simulink model "Simulink"  (R2020b)
settings: Solver=VariableStepAuto  StartTime=0.0  StopTime=11.2395  RelTol=1e-3
values from neighbouring files (symbols this model uses):
  alpha_0 = 1    [Main.m]
  b = 10    [Main.m]
  beta = 3    [Main.m]
  beta_0 = 1    [Main.m]
  c1 = rand(8,8)-0.5    [Main.m]
  c2 = rand(8,8)-0.5    [Main.m]
  c3 = rand(8,8)-0.5    [Main.m]
  c4 = rand(8,8)-0.5    [Main.m]
  delta_0 = 1    [Main.m]
  Gamma = 3    [Main.m]
  gamma = 0.1    [Main.m]
  h1_x = 5    [Main.m]
  h1_y = 5    [Main.m]
  h2_x = -5    [Main.m]
  h2_y = 5    [Main.m]
  h3_x = -5    [Main.m]
  h3_y = -5    [Main.m]
  h4_x = 5    [Main.m]
  h4_y = -5    [Main.m]
  kapa = 3    [Main.m]
  ki = diag([150,150])    [Main.m]
  kp = 20    [Main.m]
  L = full(laplacian(G))    [Main.m]
  m = 3    [Main.m]
  obs_x = 40    [Main.m]
  obs_y = 0    [Main.m]
  R = 5    [Main.m]
  r = 2    [Main.m]
  R_reg = 15    [Main.m]
  region_x = 80    [Main.m]
  region_y = 0    [Main.m]
  row_0 = 0    [Main.m]
  WL_0 = rand(number_of_neurons,1)*2    [Main.m]
  WR_0 = rand(number_of_neurons,1)*2    [Main.m]
  x1_0 = 1    [Main.m]
  x1_dot_0 = 0    [Main.m]
  x2_0 = 1    [Main.m]
  x2_dot_0 = 0    [Main.m]
  x3_0 = 1    [Main.m]
  x3_dot_0 = 0    [Main.m]
  x4_0 = 1    [Main.m]
  x4_dot_0 = 0    [Main.m]
  y1_0 = 9    [Main.m]
  y1_dot_0 = 0    [Main.m]
  y2_0 = 3    [Main.m]
  y2_dot_0 = 0    [Main.m]
  y3_0 = -3    [Main.m]
  y3_dot_0 = 0    [Main.m]
  y4_0 = -9    [Main.m]
  y4_dot_0 = 0    [Main.m]
(part 1 of 2)
settings Model: Creator=sokra  LastModifiedBy=sokra

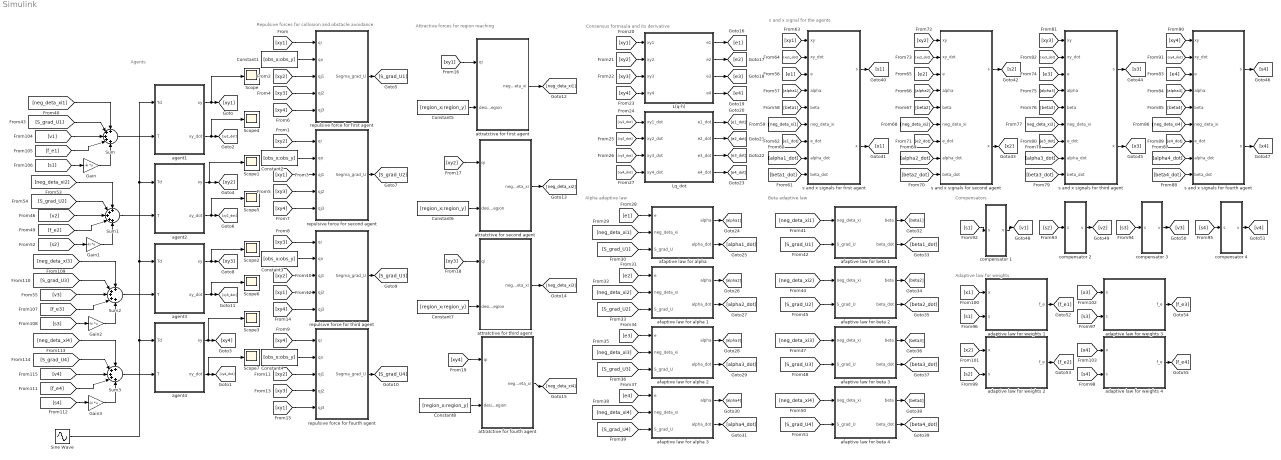
== system Simulink ==
  note: Adaptive law for weights
  note: Compensators
  note: s and x signal for the agents
  note: Alpha adaptive law
  note: Consensus formaula and its derivative
  note: Attractive forces for region reaching
  note: Repulsive forces for collosion and obstacle avoidance
  note: Agents
  note: Beta adaptive law
  Constant{1..4} (4 alike) : Constant  Value=[obs_x;obs_y]
  Constant{5..8} (4 alike) : Constant  Value=[region_x;region_y]
  Gain{,1..3} (4 alike) : Gain  Gain=-ki  Multiplication=Matrix(K*u)
  L(q-h) : Subsystem
  Lq_dot : Subsystem
  Scope{,1..7} (8 alike) : Scope
  Sine Wave : Sin  Amplitude=2  Frequency=[1;2]  Phase=[0;pi/2]  SampleTime=0
  Sum{,1..3} (4 alike) : Sum  Inputs=+++++
  adaptive law for weights 1 : Subsystem  mask{c=c1}
  adaptive law for weights 2 : Subsystem  mask{c=c2}
  adaptive law for weights 3 : Subsystem  mask{c=c3}
  adaptive law for weights 4 : Subsystem  mask{c=c4}
  "afaptive law for alpha " : Subsystem
  afaptive law for alpha 1 : Subsystem
  afaptive law for alpha 2 : Subsystem
  afaptive law for alpha 3 : Subsystem
  afaptive law for beta 1 : Subsystem
  afaptive law for beta 2 : Subsystem
  afaptive law for beta 3 : Subsystem
  afaptive law for beta 4 : Subsystem
  agent1 : Subsystem  mask{agent_x_0=x1_0, agent_y_0=y1_0, agent_x_dot_0=x1_dot_0, agent_y_dot_0=y1_dot_0}
  agent2 : Subsystem  mask{agent_x_0=x2_0, agent_y_0=y2_0, agent_x_dot_0=x2_dot_0, agent_y_dot_0=y2_dot_0}
  agent3 : Subsystem  mask{agent_x_0=x3_0, agent_y_0=y3_0, agent_x_dot_0=x3_dot_0, agent_y_dot_0=y3_dot_0}
  agent4 : Subsystem  mask{agent_x_0=x4_0, agent_y_0=y4_0, agent_x_dot_0=x4_dot_0, agent_y_dot_0=y4_dot_0}
  attratctive for first agent : Subsystem
  attratctive for fourth agent : Subsystem
  attratctive for second agent : Subsystem
  attratctive for third agent : Subsystem
  compensator 1 : Subsystem
  compensator 2 : Subsystem
  compensator 3 : Subsystem
  compensator 4 : Subsystem
  repulsive force for first agent : Subsystem
  repulsive force for fourth agent : Subsystem
  repulsive force for second agent : Subsystem
  repulsive force for third agent : Subsystem
  s and x signals for first agent : Subsystem
  s and x signals for fourth agent : Subsystem
  s and x signals for second agent : Subsystem
  s and x signals for third agent : Subsystem
  wires:
  Sine Wave/1 -> agent3/1(Td), agent2/1(Td), agent1/1(Td), agent4/1(Td)
  agent1/1(xy) -> Scope/1, [xy1]
  agent1/2(xy_dot) -> Scope4/1, [xy1_dot]
  agent2/1(xy) -> Scope1/1, [xy2]
  agent2/2(xy_dot) -> Scope5/1, [xy2_dot]
  agent3/1(xy) -> Scope2/1, [xy3]
  agent3/2(xy_dot) -> Scope6/1, [xy3_dot]
  agent4/1(xy) -> Scope3/1, [xy4]
  agent4/2(xy_dot) -> Scope7/1, [xy4_dot]
  [xy1] -> repulsive force for first agent/1(qi)
  Constant1/1 -> repulsive force for first agent/2(qo)
  [xy2] -> repulsive force for first agent/3(qj1)
  [xy3] -> repulsive force for first agent/4(qj2)
  [xy4] -> repulsive force for first agent/5(qj3)
  [xy4] -> repulsive force for second agent/5(qj3)
  [xy3] -> repulsive force for second agent/4(qj2)
  [xy1] -> repulsive force for second agent/3(qj1)
  Constant2/1 -> repulsive force for second agent/2(qo)
  [xy2] -> repulsive force for second agent/1(qi)
  [xy4] -> repulsive force for fourth agent/1(qi)
  Constant4/1 -> repulsive force for fourth agent/2(qo)
  [xy2] -> repulsive force for fourth agent/3(qj1)
  [xy3] -> repulsive force for fourth agent/4(qj2)
  [xy1] -> repulsive force for fourth agent/5(qj3)
  [xy4] -> repulsive force for third agent/5(qj3)
  [xy1] -> repulsive force for third agent/4(qj2)
  [xy2] -> repulsive force for third agent/3(qj1)
  Constant3/1 -> repulsive force for third agent/2(qo)
  [xy3] -> repulsive force for third agent/1(qi)
  repulsive force for first agent/1(Segma_grad_U) -> [S_grad_U1]
  repulsive force for second agent/1(Segma_grad_U) -> [S_grad_U2]
  repulsive force for fourth agent/1(Segma_grad_U) -> [S_grad_U4]
  repulsive force for third agent/1(Segma_grad_U) -> [S_grad_U3]
  attratctive for first agent/1(neg_deta_xi) -> [neg_deta_xi1]
  [xy1] -> attratctive for first agent/1(qi)
  Constant5/1 -> attratctive for first agent/2(desired_region)
  Constant6/1 -> attratctive for second agent/2(desired_region)
  [xy2] -> attratctive for second agent/1(qi)
  attratctive for second agent/1(neg_deta_xi) -> [neg_deta_xi2]
  attratctive for fourth agent/1(neg_deta_xi) -> [neg_deta_xi4]
  [xy4] -> attratctive for fourth agent/1(qi)
  Constant8/1 -> attratctive for fourth agent/2(desired_region)
  Constant7/1 -> attratctive for third agent/2(desired_region)
  [xy3] -> attratctive for third agent/1(qi)
  attratctive for third agent/1(neg_deta_xi) -> [neg_deta_xi3]
  [xy1] -> L(q-h)/1(xy1)
  [xy2] -> L(q-h)/2(xy2)
  [xy3] -> L(q-h)/3(xy3)
  [xy4] -> L(q-h)/4(xy4)
  L(q-h)/4(e4) -> [e4]
  L(q-h)/3(e3) -> [e3]
  L(q-h)/2(e2) -> [e2]
  L(q-h)/1(e1) -> [e1]
  Lq_dot/1(e1_dot) -> [e1_dot]
  Lq_dot/2(e2_dot) -> [e2_dot]
  Lq_dot/3(e3_dot) -> [e3_dot]
  Lq_dot/4(e4_dot) -> [e4_dot]
  [xy4_dot] -> Lq_dot/4(xy4_dot)
  [xy3_dot] -> Lq_dot/3(xy3_dot)
  [xy2_dot] -> Lq_dot/2(xy2_dot)
  [xy1_dot] -> Lq_dot/1(xy1_dot)
  [e1] -> "afaptive law for alpha "/1(e)
  [neg_deta_xi1] -> "afaptive law for alpha "/2(neg_deta_xi)
  [S_grad_U1] -> "afaptive law for alpha "/3(S_grad_U)
  "afaptive law for alpha "/1(alpha) -> [alpha1]
  "afaptive law for alpha "/2(alpha_dot) -> [alpha1_dot]
  afaptive law for alpha 1/2(alpha_dot) -> [alpha2_dot]
  afaptive law for alpha 1/1(alpha) -> [alpha2]
  [S_grad_U2] -> afaptive law for alpha 1/3(S_grad_U)
  [neg_deta_xi2] -> afaptive law for alpha 1/2(neg_deta_xi)
  [e2] -> afaptive law for alpha 1/1(e)
  [e3] -> afaptive law for alpha 2/1(e)
  [neg_deta_xi3] -> afaptive law for alpha 2/2(neg_deta_xi)
  [S_grad_U3] -> afaptive law for alpha 2/3(S_grad_U)
  afaptive law for alpha 2/1(alpha) -> [alpha3]
  afaptive law for alpha 2/2(alpha_dot) -> [alpha3_dot]
  afaptive law for alpha 3/2(alpha_dot) -> [alpha4_dot]
  afaptive law for alpha 3/1(alpha) -> [alpha4]
  [S_grad_U4] -> afaptive law for alpha 3/3(S_grad_U)
  [neg_deta_xi4] -> afaptive law for alpha 3/2(neg_deta_xi)
  [e4] -> afaptive law for alpha 3/1(e)
  [neg_deta_xi4] -> afaptive law for beta 4/1(neg_deta_xi)
  [S_grad_U4] -> afaptive law for beta 4/2(S_grad_U)
  afaptive law for beta 4/1(beta) -> [beta4]
  afaptive law for beta 4/2(beta_dot) -> [beta4_dot]
  afaptive law for beta 3/2(beta_dot) -> [beta3_dot]
  afaptive law for beta 3/1(beta) -> [beta3]
  [S_grad_U3] -> afaptive law for beta 3/2(S_grad_U)
  [neg_deta_xi3] -> afaptive law for beta 3/1(neg_deta_xi)
  [neg_deta_xi2] -> afaptive law for beta 2/1(neg_deta_xi)
  [S_grad_U2] -> afaptive law for beta 2/2(S_grad_U)
  afaptive law for beta 2/1(beta) -> [beta2]
  afaptive law for beta 2/2(beta_dot) -> [beta2_dot]
  afaptive law for beta 1/2(beta_dot) -> [beta1_dot]
  afaptive law for beta 1/1(beta) -> [beta1]
  [S_grad_U1] -> afaptive law for beta 1/2(S_grad_U)
  [neg_deta_xi1] -> afaptive law for beta 1/1(neg_deta_xi)
  Sum/1 -> agent1/2(T)
  s and x signals for first agent/2(x) -> [x1]
  s and x signals for first agent/1(s) -> [s1]
  [xy1] -> s and x signals for first agent/1(xy)
  [xy1_dot] -> s and x signals for first agent/2(xy_dot)
  [e1] -> s and x signals for first agent/3(e)
  [alpha1] -> s and x signals for first agent/4(alpha)
  [beta1] -> s and x signals for first agent/5(beta)
  [neg_deta_xi1] -> s and x signals for first agent/6(neg_deta_xi)
  [e1_dot] -> s and x signals for first agent/7(e_dot)
  [alpha1_dot] -> s and x signals for first agent/8(alpha_dot)
  [beta1_dot] -> s and x signals for first agent/9(beta_dot)
  [beta2_dot] -> s and x signals for second agent/9(beta_dot)
  [alpha2_dot] -> s and x signals for second agent/8(alpha_dot)
  [e2_dot] -> s and x signals for second agent/7(e_dot)
  [neg_deta_xi2] -> s and x signals for second agent/6(neg_deta_xi)
  [beta2] -> s and x signals for second agent/5(beta)
  [alpha2] -> s and x signals for second agent/4(alpha)
  [e2] -> s and x signals for second agent/3(e)
  [xy2_dot] -> s and x signals for second agent/2(xy_dot)
  [xy2] -> s and x signals for second agent/1(xy)
  s and x signals for second agent/1(s) -> [s2]
  s and x signals for second agent/2(x) -> [x2]
  s and x signals for third agent/2(x) -> [x3]
  s and x signals for third agent/1(s) -> [s3]
  [xy3] -> s and x signals for third agent/1(xy)
  [xy3_dot] -> s and x signals for third agent/2(xy_dot)
  [e3] -> s and x signals for third agent/3(e)
  [alpha3] -> s and x signals for third agent/4(alpha)
  [beta3] -> s and x signals for third agent/5(beta)
  [neg_deta_xi3] -> s and x signals for third agent/6(neg_deta_xi)
  [e3_dot] -> s and x signals for third agent/7(e_dot)
  [alpha3_dot] -> s and x signals for third agent/8(alpha_dot)
  [beta3_dot] -> s and x signals for third agent/9(beta_dot)
  [beta4_dot] -> s and x signals for fourth agent/9(beta_dot)
  [alpha4_dot] -> s and x signals for fourth agent/8(alpha_dot)
  [e4_dot] -> s and x signals for fourth agent/7(e_dot)
  [neg_deta_xi4] -> s and x signals for fourth agent/6(neg_deta_xi)
  [beta4] -> s and x signals for fourth agent/5(beta)
  [alpha4] -> s and x signals for fourth agent/4(alpha)
  [e4] -> s and x signals for fourth agent/3(e)
  [xy4_dot] -> s and x signals for fourth agent/2(xy_dot)
  [xy4] -> s and x signals for fourth agent/1(xy)
  s and x signals for fourth agent/1(s) -> [s4]
  s and x signals for fourth agent/2(x) -> [x4]
  [s1] -> compensator 1/1(s)
  compensator 1/1(v) -> [v1]
  compensator 2/1(v) -> [v2]
  [s2] -> compensator 2/1(s)
  [s3] -> compensator 3/1(s)
  compensator 3/1(v) -> [v3]
  compensator 4/1(v) -> [v4]
  [s4] -> compensator 4/1(s)
  [s4] -> adaptive law for weights 4/2(s)
  [s1] -> adaptive law for weights 1/2(s)
  [s3] -> adaptive law for weights 3/2(s)
  [s2] -> adaptive law for weights 2/2(s)
  [x4] -> adaptive law for weights 4/1(x)
  [x3] -> adaptive law for weights 3/1(x)
  [x2] -> adaptive law for weights 2/1(x)
  [x1] -> adaptive law for weights 1/1(x)
  adaptive law for weights 3/1(f_e) -> [f_e3]
  adaptive law for weights 4/1(f_e) -> [f_e4]
  adaptive law for weights 1/1(f_e) -> [f_e1]
  adaptive law for weights 2/1(f_e) -> [f_e2]
  [s1] -> Gain/1
  [neg_deta_xi1] -> Sum/1
  [S_grad_U1] -> Sum/2
  [v1] -> Sum/3
  [f_e1] -> Sum/4
  Gain/1 -> Sum/5
  Gain1/1 -> Sum1/5
  [f_e2] -> Sum1/4
  [v2] -> Sum1/3
  [S_grad_U2] -> Sum1/2
  [neg_deta_xi2] -> Sum1/1
  [s2] -> Gain1/1
  Sum1/1 -> agent2/2(T)
  Sum2/1 -> agent3/2(T)
  [s3] -> Gain2/1
  [neg_deta_xi3] -> Sum2/1
  [S_grad_U3] -> Sum2/2
  [v3] -> Sum2/3
  [f_e3] -> Sum2/4
  Gain2/1 -> Sum2/5
  Gain3/1 -> Sum3/5
  [f_e4] -> Sum3/4
  [v4] -> Sum3/3
  [S_grad_U4] -> Sum3/2
  [neg_deta_xi4] -> Sum3/1
  [s4] -> Gain3/1
  Sum3/1 -> agent4/2(T)

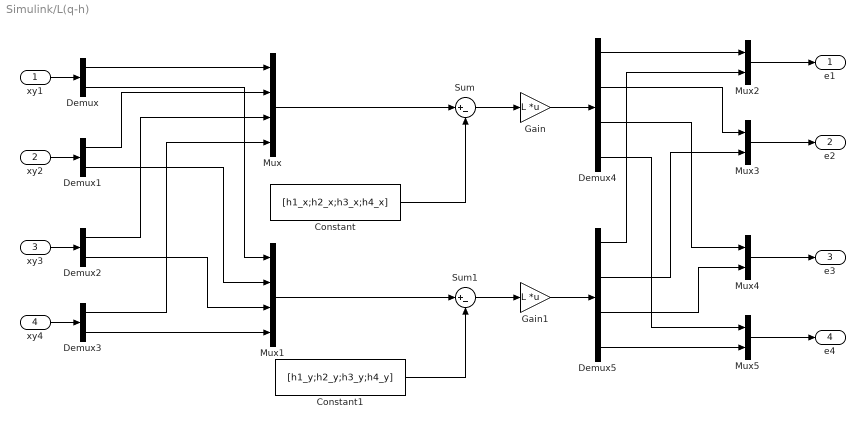
== system Simulink/L(q-h) ==
  xy1 : Inport
  xy2 : Inport  Port=2
  xy3 : Inport  Port=3
  xy4 : Inport  Port=4
  Constant : Constant  Value=[h1_x;h2_x;h3_x;h4_x]
  Constant1 : Constant  Value=[h1_y;h2_y;h3_y;h4_y]
  Demux{,1..3} (4 alike) : Demux  Outputs=2
  Demux4 : Demux
  Demux5 : Demux
  Gain : Gain  Gain=L  Multiplication=Matrix(K*u)
  Gain1 : Gain  Gain=L  Multiplication=Matrix(K*u)
  Mux : Mux
  Mux1 : Mux
  Mux{2..5} (4 alike) : Mux  Inputs=2
  Sum : Sum  Inputs=|+-
  Sum1 : Sum  Inputs=|+-
  e1 : Outport
  e2 : Outport  Port=2
  e3 : Outport  Port=3
  e4 : Outport  Port=4
  wires:
  xy1/1 -> Demux/1
  xy2/1 -> Demux1/1
  xy3/1 -> Demux2/1
  xy4/1 -> Demux3/1
  Demux/1 -> Mux/1
  Demux1/1 -> Mux/2
  Demux2/1 -> Mux/3
  Demux3/1 -> Mux/4
  Demux/2 -> Mux1/1
  Demux1/2 -> Mux1/2
  Demux2/2 -> Mux1/3
  Demux3/2 -> Mux1/4
  Mux/1 -> Sum/1
  Constant/1 -> Sum/2
  Mux1/1 -> Sum1/1
  Constant1/1 -> Sum1/2
  Sum/1 -> Gain/1
  Sum1/1 -> Gain1/1
  Gain/1 -> Demux4/1
  Gain1/1 -> Demux5/1
  Mux5/1 -> e4/1
  Mux4/1 -> e3/1
  Mux3/1 -> e2/1
  Mux2/1 -> e1/1
  Demux4/1 -> Mux2/1
  Demux4/2 -> Mux3/1
  Demux4/3 -> Mux4/1
  Demux4/4 -> Mux5/1
  Demux5/4 -> Mux5/2
  Demux5/3 -> Mux4/2
  Demux5/2 -> Mux3/2
  Demux5/1 -> Mux2/2

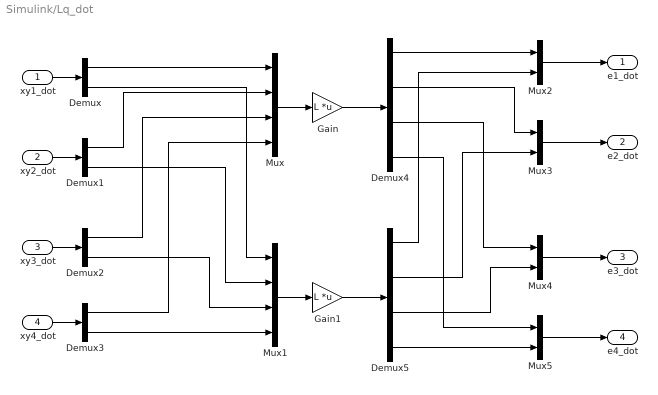
== system Simulink/Lq_dot ==
  xy1_dot : Inport
  xy2_dot : Inport  Port=2
  xy3_dot : Inport  Port=3
  xy4_dot : Inport  Port=4
  Demux{,1..3} (4 alike) : Demux  Outputs=2
  Demux4 : Demux
  Demux5 : Demux
  Gain : Gain  Gain=L  Multiplication=Matrix(K*u)
  Gain1 : Gain  Gain=L  Multiplication=Matrix(K*u)
  Mux : Mux
  Mux1 : Mux
  Mux{2..5} (4 alike) : Mux  Inputs=2
  e1_dot : Outport
  e2_dot : Outport  Port=2
  e3_dot : Outport  Port=3
  e4_dot : Outport  Port=4
  wires:
  Demux5/1 -> Mux2/2
  Demux5/2 -> Mux3/2
  Demux5/3 -> Mux4/2
  Demux5/4 -> Mux5/2
  Demux4/4 -> Mux5/1
  Demux4/3 -> Mux4/1
  Demux4/2 -> Mux3/1
  Demux4/1 -> Mux2/1
  Mux2/1 -> e1_dot/1
  Mux3/1 -> e2_dot/1
  Mux4/1 -> e3_dot/1
  Mux5/1 -> e4_dot/1
  Gain1/1 -> Demux5/1
  Gain/1 -> Demux4/1
  Mux1/1 -> Gain1/1
  Demux3/2 -> Mux1/4
  Demux2/2 -> Mux1/3
  Demux1/2 -> Mux1/2
  Demux/2 -> Mux1/1
  Demux3/1 -> Mux/4
  Demux2/1 -> Mux/3
  Demux1/1 -> Mux/2
  Demux/1 -> Mux/1
  xy4_dot/1 -> Demux3/1
  xy3_dot/1 -> Demux2/1
  xy2_dot/1 -> Demux1/1
  xy1_dot/1 -> Demux/1
  Mux/1 -> Gain/1

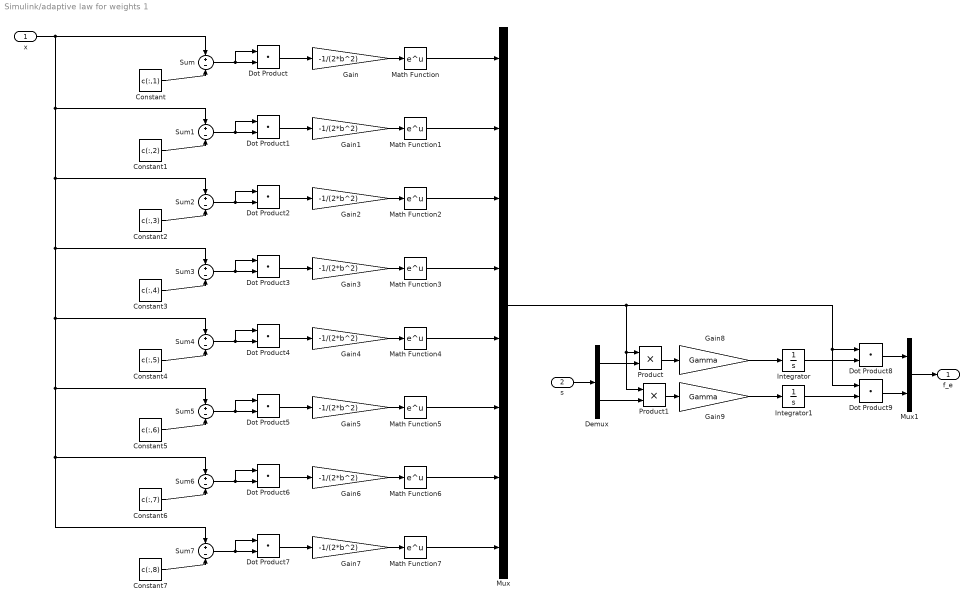
== system Simulink/adaptive law for weights 1 ==
  x : Inport
  s : Inport  Port=2
  Constant : Constant  Value=c(:,1)
  Constant1 : Constant  Value=c(:,2)
  Constant2 : Constant  Value=c(:,3)
  Constant3 : Constant  Value=c(:,4)
  Constant4 : Constant  Value=c(:,5)
  Constant5 : Constant  Value=c(:,6)
  Constant6 : Constant  Value=c(:,7)
  Constant7 : Constant  Value=c(:,8)
  Demux : Demux  Outputs=2
  Dot Product{,1..9} (10 alike) : DotProduct  InputSameDT=on  OutDataTypeStr=Inherit: Inherit via internal rule
  Gain{,1..7} (8 alike) : Gain  Gain=-1/(2*b^2)
  Gain8 : Gain  Gain=Gamma
  Gain9 : Gain  Gain=Gamma
  Integrator : Integrator  InitialCondition=WL_0
  Integrator1 : Integrator  InitialCondition=WR_0
  Math Function{,1..7} (8 alike) : Math  SaturateOnIntegerOverflow=on
  Mux : Mux  Inputs=8
  Mux1 : Mux  Inputs=2
  Product : Product
  Product1 : Product
  Sum{,1..7} (8 alike) : Sum  Inputs=+-
  f_e : Outport
  wires:
  Constant/1 -> Sum/2
  Sum/1 -> Dot Product/2, Dot Product/1
  Dot Product/1 -> Gain/1
  Gain/1 -> Math Function/1
  Math Function/1 -> Mux/1
  Math Function1/1 -> Mux/2
  Gain1/1 -> Math Function1/1
  Dot Product1/1 -> Gain1/1
  Sum1/1 -> Dot Product1/1, Dot Product1/2
  Constant1/1 -> Sum1/2
  Constant2/1 -> Sum2/2
  Sum2/1 -> Dot Product2/2, Dot Product2/1
  Dot Product2/1 -> Gain2/1
  Gain2/1 -> Math Function2/1
  Math Function2/1 -> Mux/3
  Math Function3/1 -> Mux/4
  Gain3/1 -> Math Function3/1
  Dot Product3/1 -> Gain3/1
  Sum3/1 -> Dot Product3/1, Dot Product3/2
  Constant3/1 -> Sum3/2
  Constant4/1 -> Sum4/2
  Sum4/1 -> Dot Product4/2, Dot Product4/1
  Dot Product4/1 -> Gain4/1
  Gain4/1 -> Math Function4/1
  Math Function4/1 -> Mux/5
  Math Function5/1 -> Mux/6
  Gain5/1 -> Math Function5/1
  Dot Product5/1 -> Gain5/1
  Sum5/1 -> Dot Product5/1, Dot Product5/2
  Constant5/1 -> Sum5/2
  Constant6/1 -> Sum6/2
  Sum6/1 -> Dot Product6/2, Dot Product6/1
  Dot Product6/1 -> Gain6/1
  Gain6/1 -> Math Function6/1
  Math Function6/1 -> Mux/7
  Math Function7/1 -> Mux/8
  Gain7/1 -> Math Function7/1
  Dot Product7/1 -> Gain7/1
  Sum7/1 -> Dot Product7/1, Dot Product7/2
  Constant7/1 -> Sum7/2
  x/1 -> Sum7/1, Sum6/1, Sum5/1, Sum4/1, Sum3/1, Sum2/1, Sum1/1, Sum/1
  s/1 -> Demux/1
  Mux/1 -> Dot Product9/1, Dot Product8/1, Product1/1, Product/1
  Demux/1 -> Product/2
  Demux/2 -> Product1/2
  Product/1 -> Gain8/1
  Product1/1 -> Gain9/1
  Gain8/1 -> Integrator/1
  Gain9/1 -> Integrator1/1
  Integrator1/1 -> Dot Product9/2
  Integrator/1 -> Dot Product8/2
  Dot Product8/1 -> Mux1/1
  Dot Product9/1 -> Mux1/2
  Mux1/1 -> f_e/1

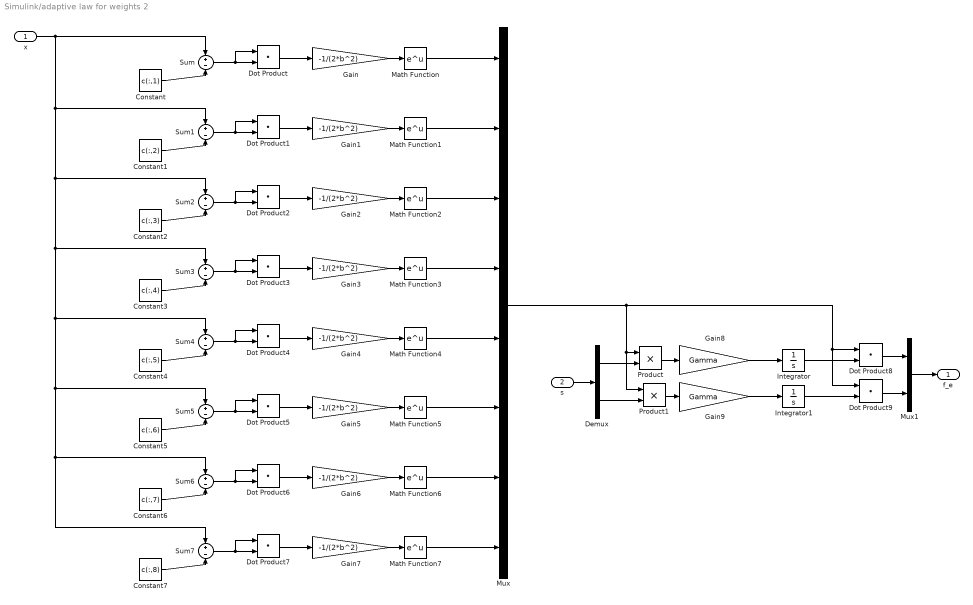
== system Simulink/adaptive law for weights 2 ==
  x : Inport
  s : Inport  Port=2
  Constant : Constant  Value=c(:,1)
  Constant1 : Constant  Value=c(:,2)
  Constant2 : Constant  Value=c(:,3)
  Constant3 : Constant  Value=c(:,4)
  Constant4 : Constant  Value=c(:,5)
  Constant5 : Constant  Value=c(:,6)
  Constant6 : Constant  Value=c(:,7)
  Constant7 : Constant  Value=c(:,8)
  Demux : Demux  Outputs=2
  Dot Product{,1..9} (10 alike) : DotProduct  InputSameDT=on  OutDataTypeStr=Inherit: Inherit via internal rule
  Gain{,1..7} (8 alike) : Gain  Gain=-1/(2*b^2)
  Gain8 : Gain  Gain=Gamma
  Gain9 : Gain  Gain=Gamma
  Integrator : Integrator  InitialCondition=WL_0
  Integrator1 : Integrator  InitialCondition=WR_0
  Math Function{,1..7} (8 alike) : Math  SaturateOnIntegerOverflow=on
  Mux : Mux  Inputs=8
  Mux1 : Mux  Inputs=2
  Product : Product
  Product1 : Product
  Sum{,1..7} (8 alike) : Sum  Inputs=+-
  f_e : Outport
  wires:
  Mux1/1 -> f_e/1
  Gain9/1 -> Integrator1/1
  Dot Product9/1 -> Mux1/2
  Integrator1/1 -> Dot Product9/2
  Math Function3/1 -> Mux/4
  Math Function7/1 -> Mux/8
  Math Function1/1 -> Mux/2
  Math Function5/1 -> Mux/6
  Math Function2/1 -> Mux/3
  Math Function6/1 -> Mux/7
  Constant7/1 -> Sum7/2
  Sum7/1 -> Dot Product7/1, Dot Product7/2
  Dot Product7/1 -> Gain7/1
  Constant3/1 -> Sum3/2
  Sum3/1 -> Dot Product3/1, Dot Product3/2
  Dot Product3/1 -> Gain3/1
  Gain3/1 -> Math Function3/1
  Constant5/1 -> Sum5/2
  Gain5/1 -> Math Function5/1
  Sum1/1 -> Dot Product1/1, Dot Product1/2
  Sum6/1 -> Dot Product6/2, Dot Product6/1
  Dot Product6/1 -> Gain6/1
  Product/1 -> Gain8/1
  Gain/1 -> Math Function/1
  Math Function/1 -> Mux/1
  Constant6/1 -> Sum6/2
  Math Function4/1 -> Mux/5
  Product1/1 -> Gain9/1
  Dot Product4/1 -> Gain4/1
  Sum4/1 -> Dot Product4/2, Dot Product4/1
  Constant4/1 -> Sum4/2
  x/1 -> Sum7/1, Sum6/1, Sum5/1, Sum4/1, Sum3/1, Sum2/1, Sum1/1, Sum/1
  Gain6/1 -> Math Function6/1
  Sum5/1 -> Dot Product5/1, Dot Product5/2
  s/1 -> Demux/1
  Demux/1 -> Product/2
  Mux/1 -> Dot Product9/1, Dot Product8/1, Product1/1, Product/1
  Gain8/1 -> Integrator/1
  Dot Product1/1 -> Gain1/1
  Gain7/1 -> Math Function7/1
  Sum/1 -> Dot Product/2, Dot Product/1
  Dot Product8/1 -> Mux1/1
  Gain1/1 -> Math Function1/1
  Dot Product2/1 -> Gain2/1
  Sum2/1 -> Dot Product2/2, Dot Product2/1
  Gain2/1 -> Math Function2/1
  Demux/2 -> Product1/2
  Constant1/1 -> Sum1/2
  Dot Product/1 -> Gain/1
  Dot Product5/1 -> Gain5/1
  Constant2/1 -> Sum2/2
  Gain4/1 -> Math Function4/1
  Integrator/1 -> Dot Product8/2
  Constant/1 -> Sum/2

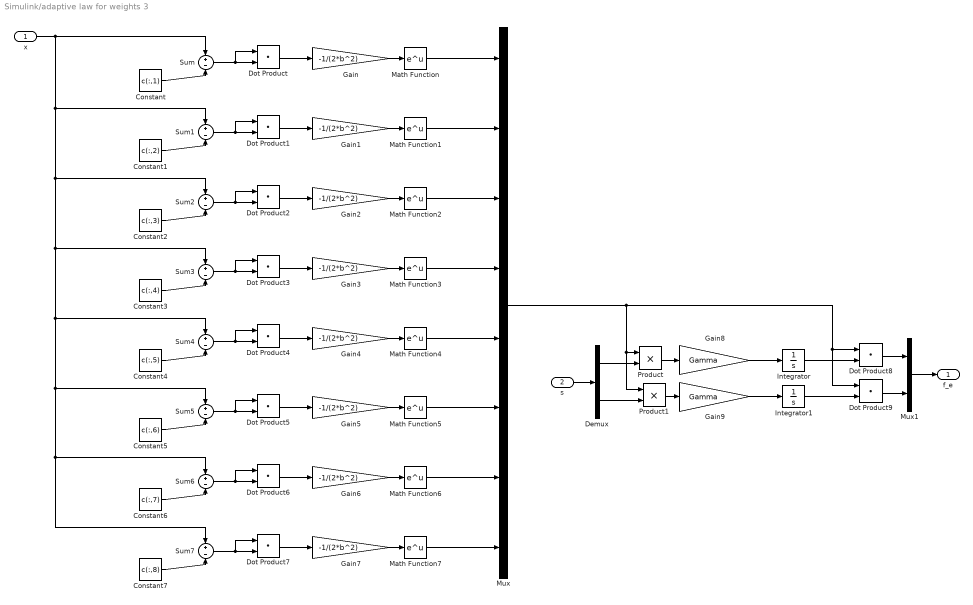
== system Simulink/adaptive law for weights 3 ==
  x : Inport
  s : Inport  Port=2
  Constant : Constant  Value=c(:,1)
  Constant1 : Constant  Value=c(:,2)
  Constant2 : Constant  Value=c(:,3)
  Constant3 : Constant  Value=c(:,4)
  Constant4 : Constant  Value=c(:,5)
  Constant5 : Constant  Value=c(:,6)
  Constant6 : Constant  Value=c(:,7)
  Constant7 : Constant  Value=c(:,8)
  Demux : Demux  Outputs=2
  Dot Product{,1..9} (10 alike) : DotProduct  InputSameDT=on  OutDataTypeStr=Inherit: Inherit via internal rule
  Gain{,1..7} (8 alike) : Gain  Gain=-1/(2*b^2)
  Gain8 : Gain  Gain=Gamma
  Gain9 : Gain  Gain=Gamma
  Integrator : Integrator  InitialCondition=WL_0
  Integrator1 : Integrator  InitialCondition=WR_0
  Math Function{,1..7} (8 alike) : Math  SaturateOnIntegerOverflow=on
  Mux : Mux  Inputs=8
  Mux1 : Mux  Inputs=2
  Product : Product
  Product1 : Product
  Sum{,1..7} (8 alike) : Sum  Inputs=+-
  f_e : Outport
  wires:
  Mux1/1 -> f_e/1
  Gain9/1 -> Integrator1/1
  Dot Product9/1 -> Mux1/2
  Integrator1/1 -> Dot Product9/2
  Math Function3/1 -> Mux/4
  Math Function7/1 -> Mux/8
  Math Function1/1 -> Mux/2
  Math Function5/1 -> Mux/6
  Math Function2/1 -> Mux/3
  Math Function6/1 -> Mux/7
  Constant7/1 -> Sum7/2
  Sum7/1 -> Dot Product7/1, Dot Product7/2
  Dot Product7/1 -> Gain7/1
  Constant3/1 -> Sum3/2
  Sum3/1 -> Dot Product3/1, Dot Product3/2
  Dot Product3/1 -> Gain3/1
  Gain3/1 -> Math Function3/1
  Constant5/1 -> Sum5/2
  Gain5/1 -> Math Function5/1
  Sum1/1 -> Dot Product1/1, Dot Product1/2
  Sum6/1 -> Dot Product6/2, Dot Product6/1
  Dot Product6/1 -> Gain6/1
  Product/1 -> Gain8/1
  Gain/1 -> Math Function/1
  Math Function/1 -> Mux/1
  Constant6/1 -> Sum6/2
  Math Function4/1 -> Mux/5
  Product1/1 -> Gain9/1
  Dot Product4/1 -> Gain4/1
  Sum4/1 -> Dot Product4/2, Dot Product4/1
  Constant4/1 -> Sum4/2
  x/1 -> Sum7/1, Sum6/1, Sum5/1, Sum4/1, Sum3/1, Sum2/1, Sum1/1, Sum/1
  Gain6/1 -> Math Function6/1
  Sum5/1 -> Dot Product5/1, Dot Product5/2
  s/1 -> Demux/1
  Demux/1 -> Product/2
  Mux/1 -> Dot Product9/1, Dot Product8/1, Product1/1, Product/1
  Gain8/1 -> Integrator/1
  Dot Product1/1 -> Gain1/1
  Gain7/1 -> Math Function7/1
  Sum/1 -> Dot Product/2, Dot Product/1
  Dot Product8/1 -> Mux1/1
  Gain1/1 -> Math Function1/1
  Dot Product2/1 -> Gain2/1
  Sum2/1 -> Dot Product2/2, Dot Product2/1
  Gain2/1 -> Math Function2/1
  Demux/2 -> Product1/2
  Constant1/1 -> Sum1/2
  Dot Product/1 -> Gain/1
  Dot Product5/1 -> Gain5/1
  Constant2/1 -> Sum2/2
  Gain4/1 -> Math Function4/1
  Integrator/1 -> Dot Product8/2
  Constant/1 -> Sum/2

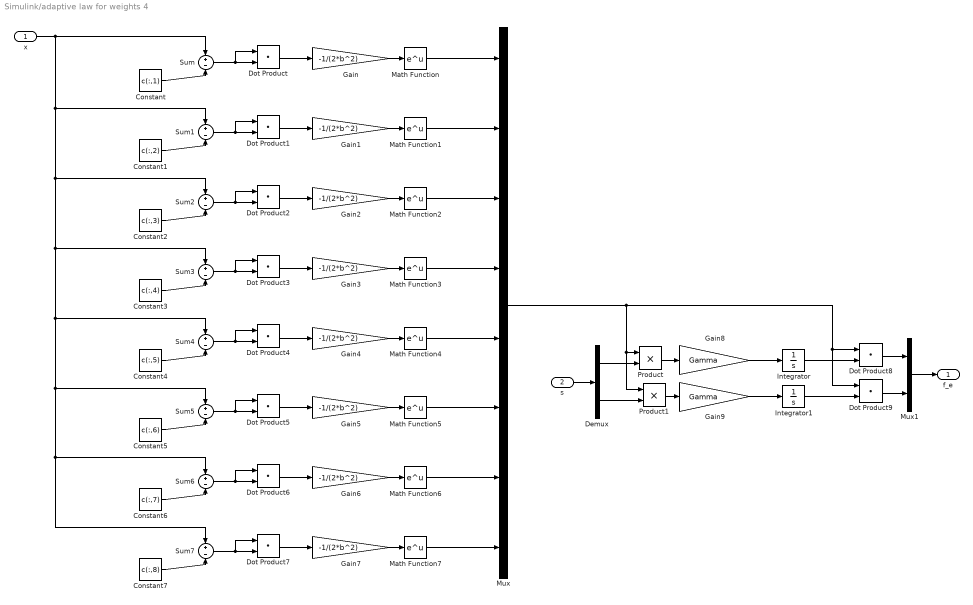
== system Simulink/adaptive law for weights 4 ==
  x : Inport
  s : Inport  Port=2
  Constant : Constant  Value=c(:,1)
  Constant1 : Constant  Value=c(:,2)
  Constant2 : Constant  Value=c(:,3)
  Constant3 : Constant  Value=c(:,4)
  Constant4 : Constant  Value=c(:,5)
  Constant5 : Constant  Value=c(:,6)
  Constant6 : Constant  Value=c(:,7)
  Constant7 : Constant  Value=c(:,8)
  Demux : Demux  Outputs=2
  Dot Product{,1..9} (10 alike) : DotProduct  InputSameDT=on  OutDataTypeStr=Inherit: Inherit via internal rule
  Gain{,1..7} (8 alike) : Gain  Gain=-1/(2*b^2)
  Gain8 : Gain  Gain=Gamma
  Gain9 : Gain  Gain=Gamma
  Integrator : Integrator  InitialCondition=WL_0
  Integrator1 : Integrator  InitialCondition=WR_0
  Math Function{,1..7} (8 alike) : Math  SaturateOnIntegerOverflow=on
  Mux : Mux  Inputs=8
  Mux1 : Mux  Inputs=2
  Product : Product
  Product1 : Product
  Sum{,1..7} (8 alike) : Sum  Inputs=+-
  f_e : Outport
  wires:
  Mux1/1 -> f_e/1
  Gain9/1 -> Integrator1/1
  Dot Product9/1 -> Mux1/2
  Integrator1/1 -> Dot Product9/2
  Math Function3/1 -> Mux/4
  Math Function7/1 -> Mux/8
  Math Function1/1 -> Mux/2
  Math Function5/1 -> Mux/6
  Math Function2/1 -> Mux/3
  Math Function6/1 -> Mux/7
  Constant7/1 -> Sum7/2
  Sum7/1 -> Dot Product7/1, Dot Product7/2
  Dot Product7/1 -> Gain7/1
  Constant3/1 -> Sum3/2
  Sum3/1 -> Dot Product3/1, Dot Product3/2
  Dot Product3/1 -> Gain3/1
  Gain3/1 -> Math Function3/1
  Constant5/1 -> Sum5/2
  Gain5/1 -> Math Function5/1
  Sum1/1 -> Dot Product1/1, Dot Product1/2
  Sum6/1 -> Dot Product6/2, Dot Product6/1
  Dot Product6/1 -> Gain6/1
  Product/1 -> Gain8/1
  Gain/1 -> Math Function/1
  Math Function/1 -> Mux/1
  Constant6/1 -> Sum6/2
  Math Function4/1 -> Mux/5
  Product1/1 -> Gain9/1
  Dot Product4/1 -> Gain4/1
  Sum4/1 -> Dot Product4/2, Dot Product4/1
  Constant4/1 -> Sum4/2
  x/1 -> Sum7/1, Sum6/1, Sum5/1, Sum4/1, Sum3/1, Sum2/1, Sum1/1, Sum/1
  Gain6/1 -> Math Function6/1
  Sum5/1 -> Dot Product5/1, Dot Product5/2
  s/1 -> Demux/1
  Demux/1 -> Product/2
  Mux/1 -> Dot Product9/1, Dot Product8/1, Product1/1, Product/1
  Gain8/1 -> Integrator/1
  Dot Product1/1 -> Gain1/1
  Gain7/1 -> Math Function7/1
  Sum/1 -> Dot Product/2, Dot Product/1
  Dot Product8/1 -> Mux1/1
  Gain1/1 -> Math Function1/1
  Dot Product2/1 -> Gain2/1
  Sum2/1 -> Dot Product2/2, Dot Product2/1
  Gain2/1 -> Math Function2/1
  Demux/2 -> Product1/2
  Constant1/1 -> Sum1/2
  Dot Product/1 -> Gain/1
  Dot Product5/1 -> Gain5/1
  Constant2/1 -> Sum2/2
  Gain4/1 -> Math Function4/1
  Integrator/1 -> Dot Product8/2
  Constant/1 -> Sum/2

== system Simulink/afaptive law for alpha  ==
  e : Inport
  neg_deta_xi : Inport  Port=2
  S_grad_U : Inport  Port=3
  Dot Product : DotProduct  InputSameDT=on  OutDataTypeStr=Inherit: Inherit via internal rule
  Gain : Gain  Gain=-1
  Integrator : Integrator  InitialCondition=alpha_0
  Product : Product
  Sum : Sum
  alpha : Outport
  alpha_dot : Outport  Port=2
  wires:
  Sum/1 -> Dot Product/2
  Product/1 -> Gain/1
  Gain/1 -> alpha_dot/1, Integrator/1
  Dot Product/1 -> Product/1
  S_grad_U/1 -> Sum/2
  e/1 -> Dot Product/1
  neg_deta_xi/1 -> Sum/1
  Integrator/1 -> alpha/1, Product/2

== system Simulink/afaptive law for alpha 1 ==
  e : Inport
  neg_deta_xi : Inport  Port=2
  S_grad_U : Inport  Port=3
  Dot Product : DotProduct  InputSameDT=on  OutDataTypeStr=Inherit: Inherit via internal rule
  Gain : Gain  Gain=-1
  Integrator : Integrator  InitialCondition=alpha_0
  Product : Product
  Sum : Sum
  alpha : Outport
  alpha_dot : Outport  Port=2
  wires:
  Integrator/1 -> Product/2, alpha/1
  neg_deta_xi/1 -> Sum/1
  e/1 -> Dot Product/1
  S_grad_U/1 -> Sum/2
  Dot Product/1 -> Product/1
  Gain/1 -> Integrator/1, alpha_dot/1
  Product/1 -> Gain/1
  Sum/1 -> Dot Product/2

== system Simulink/afaptive law for alpha 2 ==
  e : Inport
  neg_deta_xi : Inport  Port=2
  S_grad_U : Inport  Port=3
  Dot Product : DotProduct  InputSameDT=on  OutDataTypeStr=Inherit: Inherit via internal rule
  Gain : Gain  Gain=-1
  Integrator : Integrator  InitialCondition=alpha_0
  Product : Product
  Sum : Sum
  alpha : Outport
  alpha_dot : Outport  Port=2
  wires:
  Sum/1 -> Dot Product/2
  Product/1 -> Gain/1
  Gain/1 -> alpha_dot/1, Integrator/1
  Dot Product/1 -> Product/1
  S_grad_U/1 -> Sum/2
  e/1 -> Dot Product/1
  neg_deta_xi/1 -> Sum/1
  Integrator/1 -> alpha/1, Product/2

== system Simulink/afaptive law for alpha 3 ==
  e : Inport
  neg_deta_xi : Inport  Port=2
  S_grad_U : Inport  Port=3
  Dot Product : DotProduct  InputSameDT=on  OutDataTypeStr=Inherit: Inherit via internal rule
  Gain : Gain  Gain=-1
  Integrator : Integrator  InitialCondition=alpha_0
  Product : Product
  Sum : Sum
  alpha : Outport
  alpha_dot : Outport  Port=2
  wires:
  Integrator/1 -> Product/2, alpha/1
  neg_deta_xi/1 -> Sum/1
  e/1 -> Dot Product/1
  S_grad_U/1 -> Sum/2
  Dot Product/1 -> Product/1
  Gain/1 -> Integrator/1, alpha_dot/1
  Product/1 -> Gain/1
  Sum/1 -> Dot Product/2

== system Simulink/afaptive law for beta 1 ==
  neg_deta_xi : Inport
  S_grad_U : Inport  Port=2
  Dot Product : DotProduct  InputSameDT=on  OutDataTypeStr=Inherit: Inherit via internal rule
  Integrator : Integrator  InitialCondition=beta_0
  Product : Product
  beta : Outport
  beta_dot : Outport  Port=2
  wires:
  Integrator/1 -> Product/2, beta/1
  Dot Product/1 -> Product/1
  Product/1 -> Integrator/1, beta_dot/1
  neg_deta_xi/1 -> Dot Product/1
  S_grad_U/1 -> Dot Product/2

== system Simulink/afaptive law for beta 2 ==
  neg_deta_xi : Inport
  S_grad_U : Inport  Port=2
  Dot Product : DotProduct  InputSameDT=on  OutDataTypeStr=Inherit: Inherit via internal rule
  Integrator : Integrator  InitialCondition=beta_0
  Product : Product
  beta : Outport
  beta_dot : Outport  Port=2
  wires:
  neg_deta_xi/1 -> Dot Product/1
  Dot Product/1 -> Product/1
  Integrator/1 -> Product/2, beta/1
  Product/1 -> Integrator/1, beta_dot/1
  S_grad_U/1 -> Dot Product/2

== system Simulink/afaptive law for beta 3 ==
  neg_deta_xi : Inport
  S_grad_U : Inport  Port=2
  Dot Product : DotProduct  InputSameDT=on  OutDataTypeStr=Inherit: Inherit via internal rule
  Integrator : Integrator  InitialCondition=beta_0
  Product : Product
  beta : Outport
  beta_dot : Outport  Port=2
  wires:
  neg_deta_xi/1 -> Dot Product/1
  Dot Product/1 -> Product/1
  Integrator/1 -> Product/2, beta/1
  Product/1 -> Integrator/1, beta_dot/1
  S_grad_U/1 -> Dot Product/2

== system Simulink/afaptive law for beta 4 ==
  neg_deta_xi : Inport
  S_grad_U : Inport  Port=2
  Dot Product : DotProduct  InputSameDT=on  OutDataTypeStr=Inherit: Inherit via internal rule
  Integrator : Integrator  InitialCondition=beta_0
  Product : Product
  beta : Outport
  beta_dot : Outport  Port=2
  wires:
  neg_deta_xi/1 -> Dot Product/1
  Dot Product/1 -> Product/1
  Integrator/1 -> Product/2, beta/1
  Product/1 -> Integrator/1, beta_dot/1
  S_grad_U/1 -> Dot Product/2

== system Simulink/agent1 ==
  Td : Inport
  T : Inport  Port=2
  Gain1 : Gain  Gain=beta/m
  Gain2 : Gain  Gain=1/m
  Gain3 : Gain  Gain=1/m
  Integrator : Integrator  InitialCondition=[agent_x_dot_0;agent_x_dot_0]
  Integrator1 : Integrator  InitialCondition=[agent_x_0;agent_y_0]
  Sum : Sum  Inputs=-+-
  xy : Outport
  xy_dot : Outport  Port=2
  wires:
  Sum/1 -> Integrator/1
  Integrator/1 -> Gain1/1, xy_dot/1, Integrator1/1
  Gain2/1 -> Sum/2
  Gain1/1 -> Sum/3
  Gain3/1 -> Sum/1
  Td/1 -> Gain3/1
  Integrator1/1 -> xy/1
  T/1 -> Gain2/1

== system Simulink/agent2 ==
  Td : Inport
  T : Inport  Port=2
  Gain1 : Gain  Gain=beta/m
  Gain2 : Gain  Gain=1/m
  Gain3 : Gain  Gain=1/m
  Integrator : Integrator  InitialCondition=[agent_x_dot_0;agent_x_dot_0]
  Integrator1 : Integrator  InitialCondition=[agent_x_0;agent_y_0]
  Sum : Sum  Inputs=-+-
  xy : Outport
  xy_dot : Outport  Port=2
  wires:
  Integrator1/1 -> xy/1
  Gain3/1 -> Sum/1
  T/1 -> Gain2/1
  Sum/1 -> Integrator/1
  Integrator/1 -> Gain1/1, xy_dot/1, Integrator1/1
  Gain1/1 -> Sum/3
  Td/1 -> Gain3/1
  Gain2/1 -> Sum/2

== system Simulink/agent3 ==
  Td : Inport
  T : Inport  Port=2
  Gain1 : Gain  Gain=beta/m
  Gain2 : Gain  Gain=1/m
  Gain3 : Gain  Gain=1/m
  Integrator : Integrator  InitialCondition=[agent_x_dot_0;agent_x_dot_0]
  Integrator1 : Integrator  InitialCondition=[agent_x_0;agent_y_0]
  Sum : Sum  Inputs=-+-
  xy : Outport
  xy_dot : Outport  Port=2
  wires:
  Integrator1/1 -> xy/1
  Gain3/1 -> Sum/1
  T/1 -> Gain2/1
  Sum/1 -> Integrator/1
  Integrator/1 -> Gain1/1, xy_dot/1, Integrator1/1
  Gain1/1 -> Sum/3
  Td/1 -> Gain3/1
  Gain2/1 -> Sum/2

== system Simulink/agent4 ==
  Td : Inport
  T : Inport  Port=2
  Gain1 : Gain  Gain=beta/m
  Gain2 : Gain  Gain=1/m
  Gain3 : Gain  Gain=1/m
  Integrator : Integrator  InitialCondition=[agent_x_dot_0;agent_x_dot_0]
  Integrator1 : Integrator  InitialCondition=[agent_x_0;agent_y_0]
  Sum : Sum  Inputs=-+-
  xy : Outport
  xy_dot : Outport  Port=2
  wires:
  Integrator1/1 -> xy/1
  Gain3/1 -> Sum/1
  T/1 -> Gain2/1
  Sum/1 -> Integrator/1
  Integrator/1 -> Gain1/1, xy_dot/1, Integrator1/1
  Gain1/1 -> Sum/3
  Td/1 -> Gain3/1
  Gain2/1 -> Sum/2

== system Simulink/attratctive for first agent ==
  qi : Inport
  desired_region : Inport  Port=2
  Constant : Constant  Value=kp
  Constant3 : Constant  Value=R_reg^2
  Constant5 : Constant  Value=[0;0]
  Divide : Product  Inputs=*/
  Dot Product : DotProduct  InputSameDT=on  OutDataTypeStr=Inherit: Inherit via internal rule
  Product2 : Product
  Sqrt : Sqrt  SaturateOnIntegerOverflow=on
  Sum : Sum  Inputs=-+
  Sum1 : Sum  Inputs=+-
  Switch : Switch  Criteria=u2 > Threshold
  Transport Delay : TransportDelay
  neg_deta_xi : Outport
  wires:
  Switch/1 -> neg_deta_xi/1
  Constant/1 -> Product2/1
  Product2/1 -> Switch/1
  Dot Product/1 -> Sum1/1, Sqrt/1
  Constant5/1 -> Switch/3
  Divide/1 -> Product2/2
  Constant3/1 -> Sum1/2
  Sum/1 -> Dot Product/2, Divide/1, Dot Product/1
  Sqrt/1 -> Divide/2
  desired_region/1 -> Sum/2
  qi/1 -> Sum/1
  Sum1/1 -> Transport Delay/1
  Transport Delay/1 -> Switch/2

== system Simulink/attratctive for fourth agent ==
  qi : Inport
  desired_region : Inport  Port=2
  Constant : Constant  Value=kp
  Constant3 : Constant  Value=R_reg^2
  Constant5 : Constant  Value=[0;0]
  Divide : Product  Inputs=*/
  Dot Product : DotProduct  InputSameDT=on  OutDataTypeStr=Inherit: Inherit via internal rule
  Product2 : Product
  Sqrt : Sqrt  SaturateOnIntegerOverflow=on
  Sum : Sum  Inputs=-+
  Sum1 : Sum  Inputs=+-
  Switch : Switch  Criteria=u2 > Threshold
  Transport Delay : TransportDelay
  neg_deta_xi : Outport
  wires:
  Switch/1 -> neg_deta_xi/1
  Constant/1 -> Product2/1
  Product2/1 -> Switch/1
  qi/1 -> Sum/1
  Dot Product/1 -> Sum1/1, Sqrt/1
  Constant5/1 -> Switch/3
  Divide/1 -> Product2/2
  Constant3/1 -> Sum1/2
  Sum/1 -> Dot Product/2, Divide/1, Dot Product/1
  desired_region/1 -> Sum/2
  Sqrt/1 -> Divide/2
  Sum1/1 -> Transport Delay/1
  Transport Delay/1 -> Switch/2

== system Simulink/attratctive for second agent ==
  qi : Inport
  desired_region : Inport  Port=2
  Constant : Constant  Value=kp
  Constant3 : Constant  Value=R_reg^2
  Constant5 : Constant  Value=[0;0]
  Divide : Product  Inputs=*/
  Dot Product : DotProduct  InputSameDT=on  OutDataTypeStr=Inherit: Inherit via internal rule
  Product2 : Product
  Sqrt : Sqrt  SaturateOnIntegerOverflow=on
  Sum : Sum  Inputs=-+
  Sum1 : Sum  Inputs=+-
  Switch : Switch  Criteria=u2 > Threshold
  Transport Delay : TransportDelay
  neg_deta_xi : Outport
  wires:
  Sqrt/1 -> Divide/2
  desired_region/1 -> Sum/2
  Sum/1 -> Dot Product/1, Divide/1, Dot Product/2
  Constant3/1 -> Sum1/2
  Divide/1 -> Product2/2
  Constant5/1 -> Switch/3
  Dot Product/1 -> Sqrt/1, Sum1/1
  qi/1 -> Sum/1
  Product2/1 -> Switch/1
  Constant/1 -> Product2/1
  Switch/1 -> neg_deta_xi/1
  Sum1/1 -> Transport Delay/1
  Transport Delay/1 -> Switch/2

== system Simulink/attratctive for third agent ==
  qi : Inport
  desired_region : Inport  Port=2
  Constant : Constant  Value=kp
  Constant3 : Constant  Value=R_reg^2
  Constant5 : Constant  Value=[0;0]
  Divide : Product  Inputs=*/
  Dot Product : DotProduct  InputSameDT=on  OutDataTypeStr=Inherit: Inherit via internal rule
  Product2 : Product
  Sqrt : Sqrt  SaturateOnIntegerOverflow=on
  Sum : Sum  Inputs=-+
  Sum1 : Sum  Inputs=+-
  Switch : Switch  Criteria=u2 > Threshold
  Transport Delay : TransportDelay
  neg_deta_xi : Outport
  wires:
  Sqrt/1 -> Divide/2
  desired_region/1 -> Sum/2
  Sum/1 -> Dot Product/1, Divide/1, Dot Product/2
  Constant3/1 -> Sum1/2
  Divide/1 -> Product2/2
  Constant5/1 -> Switch/3
  Dot Product/1 -> Sqrt/1, Sum1/1
  qi/1 -> Sum/1
  Product2/1 -> Switch/1
  Constant/1 -> Product2/1
  Switch/1 -> neg_deta_xi/1
  Sum1/1 -> Transport Delay/1
  Transport Delay/1 -> Switch/2

== system Simulink/compensator 1 ==
  s : Inport
  Divide : Product  Inputs=/*
  Dot Product : DotProduct  InputSameDT=on  OutDataTypeStr=Inherit: Inherit via internal rule
  Gain : Gain  Gain=kapa
  Gain1 : Gain  Gain=-gamma
  Gain2 : Gain  Gain=-1
  Integrator : Integrator  InitialCondition=row_0
  Integrator1 : Integrator  InitialCondition=delta_0
  Product : Product
  Product1 : Product
  Product2 : Product
  Sum : Sum  Inputs=++|
  v : Outport
  wires:
  s/1 -> Product2/2, Dot Product/2, Dot Product/1
  Dot Product/1 -> Product/1, Gain/1  "norm(s)"
  Gain/1 -> Integrator/1
  Integrator/1 -> Product1/1, Product1/2, Product/2  "row"
  Gain1/1 -> Integrator1/1
  Integrator1/1 -> Sum/1, Gain1/1  "delta"
  Product/1 -> Sum/2
  Product1/1 -> Product2/1
  Product2/1 -> Gain2/1
  Gain2/1 -> Divide/2
  Sum/1 -> Divide/1
  Divide/1 -> v/1

== system Simulink/compensator 2 ==
  s : Inport
  Divide : Product  Inputs=/*
  Dot Product : DotProduct  InputSameDT=on  OutDataTypeStr=Inherit: Inherit via internal rule
  Gain : Gain  Gain=kapa
  Gain1 : Gain  Gain=-gamma
  Gain2 : Gain  Gain=-1
  Integrator : Integrator  InitialCondition=row_0
  Integrator1 : Integrator  InitialCondition=delta_0
  Product : Product
  Product1 : Product
  Product2 : Product
  Sum : Sum  Inputs=++|
  v : Outport
  wires:
  Divide/1 -> v/1
  Sum/1 -> Divide/1
  Gain2/1 -> Divide/2
  Product2/1 -> Gain2/1
  Product1/1 -> Product2/1
  Product/1 -> Sum/2
  Integrator1/1 -> Gain1/1, Sum/1  "delta"
  Gain1/1 -> Integrator1/1
  Integrator/1 -> Product/2, Product1/2, Product1/1  "row"
  Gain/1 -> Integrator/1
  Dot Product/1 -> Gain/1, Product/1  "norm(s)"
  s/1 -> Dot Product/1, Dot Product/2, Product2/2

== system Simulink/compensator 3 ==
  s : Inport
  Divide : Product  Inputs=/*
  Dot Product : DotProduct  InputSameDT=on  OutDataTypeStr=Inherit: Inherit via internal rule
  Gain : Gain  Gain=kapa
  Gain1 : Gain  Gain=-gamma
  Gain2 : Gain  Gain=-1
  Integrator : Integrator  InitialCondition=row_0
  Integrator1 : Integrator  InitialCondition=delta_0
  Product : Product
  Product1 : Product
  Product2 : Product
  Sum : Sum  Inputs=++|
  v : Outport
  wires:
  s/1 -> Product2/2, Dot Product/2, Dot Product/1
  Dot Product/1 -> Product/1, Gain/1  "norm(s)"
  Gain/1 -> Integrator/1
  Integrator/1 -> Product1/1, Product1/2, Product/2  "row"
  Gain1/1 -> Integrator1/1
  Integrator1/1 -> Sum/1, Gain1/1  "delta"
  Product/1 -> Sum/2
  Product1/1 -> Product2/1
  Product2/1 -> Gain2/1
  Gain2/1 -> Divide/2
  Sum/1 -> Divide/1
  Divide/1 -> v/1

== system Simulink/compensator 4 ==
  s : Inport
  Divide : Product  Inputs=/*
  Dot Product : DotProduct  InputSameDT=on  OutDataTypeStr=Inherit: Inherit via internal rule
  Gain : Gain  Gain=kapa
  Gain1 : Gain  Gain=-gamma
  Gain2 : Gain  Gain=-1
  Integrator : Integrator  InitialCondition=row_0
  Integrator1 : Integrator  InitialCondition=delta_0
  Product : Product
  Product1 : Product
  Product2 : Product
  Sum : Sum  Inputs=++|
  v : Outport
  wires:
  Divide/1 -> v/1
  Sum/1 -> Divide/1
  Gain2/1 -> Divide/2
  Product2/1 -> Gain2/1
  Product1/1 -> Product2/1
  Product/1 -> Sum/2
  Integrator1/1 -> Gain1/1, Sum/1  "delta"
  Gain1/1 -> Integrator1/1
  Integrator/1 -> Product/2, Product1/2, Product1/1  "row"
  Gain/1 -> Integrator/1
  Dot Product/1 -> Gain/1, Product/1  "norm(s)"
  s/1 -> Dot Product/1, Dot Product/2, Product2/2

== system Simulink/repulsive force for first agent ==
  qi : Inport
  qo : Inport  Port=2
  qj1 : Inport  Port=3
  qj2 : Inport  Port=4
  qj3 : Inport  Port=5
  Collision and obstacle avoidance function : Subsystem
  Collision and obstacle avoidance function1 : Subsystem
  Collision and obstacle avoidance function2 : Subsystem
  Collision and obstacle avoidance function3 : Subsystem
  Sum : Sum  Inputs=++++
  Segma_grad_U : Outport
  wires:
  Collision and obstacle avoidance function/1(grad_U) -> Sum/1
  qi/1 -> Collision and obstacle avoidance function2/1(qi), Collision and obstacle avoidance function3/1(qi), Collision and obstacle avoidance function1/1(qi), Collision and obstacle avoidance function/1(qi)
  Collision and obstacle avoidance function3/1(grad_U) -> Sum/4
  Collision and obstacle avoidance function2/1(grad_U) -> Sum/3
  Collision and obstacle avoidance function1/1(grad_U) -> Sum/2
  qo/1 -> Collision and obstacle avoidance function/2(qo)
  qj1/1 -> Collision and obstacle avoidance function1/2(qj)
  qj3/1 -> Collision and obstacle avoidance function3/2(qj)
  qj2/1 -> Collision and obstacle avoidance function2/2(qj)
  Sum/1 -> Segma_grad_U/1

== system Simulink/repulsive force for fourth agent ==
  qi : Inport
  qo : Inport  Port=2
  qj1 : Inport  Port=3
  qj2 : Inport  Port=4
  qj3 : Inport  Port=5
  Collision and obstacle avoidance function : Subsystem
  Collision and obstacle avoidance function1 : Subsystem
  Collision and obstacle avoidance function2 : Subsystem
  Collision and obstacle avoidance function3 : Subsystem
  Sum : Sum  Inputs=++++
  Segma_grad_U : Outport
  wires:
  Collision and obstacle avoidance function/1(grad_U) -> Sum/1
  qi/1 -> Collision and obstacle avoidance function2/1(qi), Collision and obstacle avoidance function3/1(qi), Collision and obstacle avoidance function1/1(qi), Collision and obstacle avoidance function/1(qi)
  Collision and obstacle avoidance function3/1(grad_U) -> Sum/4
  Collision and obstacle avoidance function2/1(grad_U) -> Sum/3
  Collision and obstacle avoidance function1/1(grad_U) -> Sum/2
  qo/1 -> Collision and obstacle avoidance function/2(qo)
  qj1/1 -> Collision and obstacle avoidance function1/2(qj)
  qj3/1 -> Collision and obstacle avoidance function3/2(qj)
  qj2/1 -> Collision and obstacle avoidance function2/2(qj)
  Sum/1 -> Segma_grad_U/1

== system Simulink/repulsive force for second agent ==
  qi : Inport
  qo : Inport  Port=2
  qj1 : Inport  Port=3
  qj2 : Inport  Port=4
  qj3 : Inport  Port=5
  Collision and obstacle avoidance function : Subsystem
  Collision and obstacle avoidance function1 : Subsystem
  Collision and obstacle avoidance function2 : Subsystem
  Collision and obstacle avoidance function3 : Subsystem
  Sum : Sum  Inputs=++++
  Segma_grad_U : Outport
  wires:
  Sum/1 -> Segma_grad_U/1
  qj2/1 -> Collision and obstacle avoidance function2/2(qj)
  qj3/1 -> Collision and obstacle avoidance function3/2(qj)
  qj1/1 -> Collision and obstacle avoidance function1/2(qj)
  qo/1 -> Collision and obstacle avoidance function/2(qo)
  Collision and obstacle avoidance function1/1(grad_U) -> Sum/2
  Collision and obstacle avoidance function2/1(grad_U) -> Sum/3
  Collision and obstacle avoidance function3/1(grad_U) -> Sum/4
  qi/1 -> Collision and obstacle avoidance function/1(qi), Collision and obstacle avoidance function1/1(qi), Collision and obstacle avoidance function3/1(qi), Collision and obstacle avoidance function2/1(qi)
  Collision and obstacle avoidance function/1(grad_U) -> Sum/1

== system Simulink/repulsive force for third agent ==
  qi : Inport
  qo : Inport  Port=2
  qj1 : Inport  Port=3
  qj2 : Inport  Port=4
  qj3 : Inport  Port=5
  Collision and obstacle avoidance function : Subsystem
  Collision and obstacle avoidance function1 : Subsystem
  Collision and obstacle avoidance function2 : Subsystem
  Collision and obstacle avoidance function3 : Subsystem
  Sum : Sum  Inputs=++++
  Segma_grad_U : Outport
  wires:
  Sum/1 -> Segma_grad_U/1
  qj2/1 -> Collision and obstacle avoidance function2/2(qj)
  qj3/1 -> Collision and obstacle avoidance function3/2(qj)
  qj1/1 -> Collision and obstacle avoidance function1/2(qj)
  qo/1 -> Collision and obstacle avoidance function/2(qo)
  Collision and obstacle avoidance function1/1(grad_U) -> Sum/2
  Collision and obstacle avoidance function2/1(grad_U) -> Sum/3
  Collision and obstacle avoidance function3/1(grad_U) -> Sum/4
  qi/1 -> Collision and obstacle avoidance function/1(qi), Collision and obstacle avoidance function1/1(qi), Collision and obstacle avoidance function3/1(qi), Collision and obstacle avoidance function2/1(qi)
  Collision and obstacle avoidance function/1(grad_U) -> Sum/1

== system Simulink/s and x signals for first agent ==
  xy : Inport
  xy_dot : Inport  Port=2
  e : Inport  Port=3
  alpha : Inport  Port=4
  beta : Inport  Port=5
  neg_deta_xi : Inport  Port=6
  e_dot : Inport  Port=7
  alpha_dot : Inport  Port=8
  beta_dot : Inport  Port=9
  Derivative : Derivative
  Mux : Mux
  Sum : Sum  Inputs=|+-
  qri_dot : Subsystem
  qri_dot_dot : Subsystem
  s : Outport
  x : Outport  Port=2
  wires:
  e/1 -> qri_dot_dot/1(e), qri_dot/1(e)
  alpha/1 -> qri_dot_dot/2(alpha), qri_dot/2(alpha)
  beta/1 -> qri_dot_dot/3(beta), qri_dot/3(beta)
  neg_deta_xi/1 -> Derivative/1, qri_dot_dot/4(neg_deta_xi), qri_dot/4(neg_deta_xi)
  xy_dot/1 -> Mux/1, Sum/1
  qri_dot/1(qri_dot) -> Mux/4, Sum/2
  Sum/1 -> s/1
  beta_dot/1 -> qri_dot_dot/7(beta_dot)
  alpha_dot/1 -> qri_dot_dot/6(alpha_dot)
  e_dot/1 -> qri_dot_dot/5(e_dot)
  Derivative/1 -> qri_dot_dot/8(neg_deta_xi_dot)
  Mux/1 -> x/1
  xy/1 -> Mux/2
  qri_dot_dot/1(qri_dot_dot) -> Mux/3

== system Simulink/s and x signals for fourth agent ==
  xy : Inport
  xy_dot : Inport  Port=2
  e : Inport  Port=3
  alpha : Inport  Port=4
  beta : Inport  Port=5
  neg_deta_xi : Inport  Port=6
  e_dot : Inport  Port=7
  alpha_dot : Inport  Port=8
  beta_dot : Inport  Port=9
  Derivative : Derivative
  Mux : Mux
  Sum : Sum  Inputs=|+-
  qri_dot : Subsystem
  qri_dot_dot : Subsystem
  s : Outport
  x : Outport  Port=2
  wires:
  qri_dot_dot/1(qri_dot_dot) -> Mux/3
  xy/1 -> Mux/2
  Mux/1 -> x/1
  Derivative/1 -> qri_dot_dot/8(neg_deta_xi_dot)
  e_dot/1 -> qri_dot_dot/5(e_dot)
  alpha_dot/1 -> qri_dot_dot/6(alpha_dot)
  beta_dot/1 -> qri_dot_dot/7(beta_dot)
  Sum/1 -> s/1
  qri_dot/1(qri_dot) -> Sum/2, Mux/4
  xy_dot/1 -> Sum/1, Mux/1
  neg_deta_xi/1 -> qri_dot/4(neg_deta_xi), qri_dot_dot/4(neg_deta_xi), Derivative/1
  beta/1 -> qri_dot/3(beta), qri_dot_dot/3(beta)
  alpha/1 -> qri_dot/2(alpha), qri_dot_dot/2(alpha)
  e/1 -> qri_dot/1(e), qri_dot_dot/1(e)

== system Simulink/s and x signals for second agent ==
  xy : Inport
  xy_dot : Inport  Port=2
  e : Inport  Port=3
  alpha : Inport  Port=4
  beta : Inport  Port=5
  neg_deta_xi : Inport  Port=6
  e_dot : Inport  Port=7
  alpha_dot : Inport  Port=8
  beta_dot : Inport  Port=9
  Derivative : Derivative
  Mux : Mux
  Sum : Sum  Inputs=|+-
  qri_dot : Subsystem
  qri_dot_dot : Subsystem
  s : Outport
  x : Outport  Port=2
  wires:
  qri_dot_dot/1(qri_dot_dot) -> Mux/3
  xy/1 -> Mux/2
  Mux/1 -> x/1
  Derivative/1 -> qri_dot_dot/8(neg_deta_xi_dot)
  e_dot/1 -> qri_dot_dot/5(e_dot)
  alpha_dot/1 -> qri_dot_dot/6(alpha_dot)
  beta_dot/1 -> qri_dot_dot/7(beta_dot)
  Sum/1 -> s/1
  qri_dot/1(qri_dot) -> Sum/2, Mux/4
  xy_dot/1 -> Sum/1, Mux/1
  neg_deta_xi/1 -> qri_dot/4(neg_deta_xi), qri_dot_dot/4(neg_deta_xi), Derivative/1
  beta/1 -> qri_dot/3(beta), qri_dot_dot/3(beta)
  alpha/1 -> qri_dot/2(alpha), qri_dot_dot/2(alpha)
  e/1 -> qri_dot/1(e), qri_dot_dot/1(e)

== system Simulink/s and x signals for third agent ==
  xy : Inport
  xy_dot : Inport  Port=2
  e : Inport  Port=3
  alpha : Inport  Port=4
  beta : Inport  Port=5
  neg_deta_xi : Inport  Port=6
  e_dot : Inport  Port=7
  alpha_dot : Inport  Port=8
  beta_dot : Inport  Port=9
  Derivative : Derivative
  Mux : Mux
  Sum : Sum  Inputs=|+-
  qri_dot : Subsystem
  qri_dot_dot : Subsystem
  s : Outport
  x : Outport  Port=2
  wires:
  e/1 -> qri_dot_dot/1(e), qri_dot/1(e)
  alpha/1 -> qri_dot_dot/2(alpha), qri_dot/2(alpha)
  beta/1 -> qri_dot_dot/3(beta), qri_dot/3(beta)
  neg_deta_xi/1 -> Derivative/1, qri_dot_dot/4(neg_deta_xi), qri_dot/4(neg_deta_xi)
  xy_dot/1 -> Mux/1, Sum/1
  qri_dot/1(qri_dot) -> Mux/4, Sum/2
  Sum/1 -> s/1
  beta_dot/1 -> qri_dot_dot/7(beta_dot)
  alpha_dot/1 -> qri_dot_dot/6(alpha_dot)
  e_dot/1 -> qri_dot_dot/5(e_dot)
  Derivative/1 -> qri_dot_dot/8(neg_deta_xi_dot)
  Mux/1 -> x/1
  xy/1 -> Mux/2
  qri_dot_dot/1(qri_dot_dot) -> Mux/3

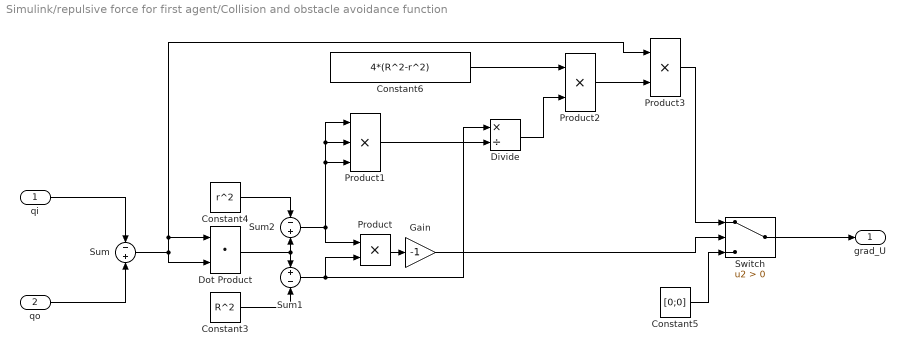
== system Simulink/repulsive force for first agent/Collision and obstacle avoidance function ==
  qi : Inport
  qo : Inport  Port=2
  Constant3 : Constant  Value=R^2
  Constant4 : Constant  Value=r^2
  Constant5 : Constant  Value=[0;0]
  Constant6 : Constant  Value=4*(R^2-r^2)
  Divide : Product  Inputs=*/
  Dot Product : DotProduct  InputSameDT=on  OutDataTypeStr=Inherit: Inherit via internal rule
  Gain : Gain  Gain=-1
  Product : Product
  Product1 : Product  Inputs=3
  Product2 : Product
  Product3 : Product
  Sum : Sum  Inputs=-+
  Sum1 : Sum  Inputs=+-
  Sum2 : Sum  Inputs=-+
  Switch : Switch  Criteria=u2 > Threshold
  grad_U : Outport
  wires:
  Sum1/1 -> Divide/1, Product/2
  Sum2/1 -> Product1/1, Product1/2, Product1/3, Product/1
  qi/1 -> Sum/1
  Dot Product/1 -> Sum2/2, Sum1/1
  Product1/1 -> Divide/2
  Constant5/1 -> Switch/3
  Constant4/1 -> Sum2/1
  Divide/1 -> Product2/2
  Constant3/1 -> Sum1/2
  Sum/1 -> Product3/1, Dot Product/1, Dot Product/2
  Product/1 -> Gain/1
  Gain/1 -> Switch/2
  Constant6/1 -> Product2/1
  Product3/1 -> Switch/1
  Product2/1 -> Product3/2
  Switch/1 -> grad_U/1
  qo/1 -> Sum/2

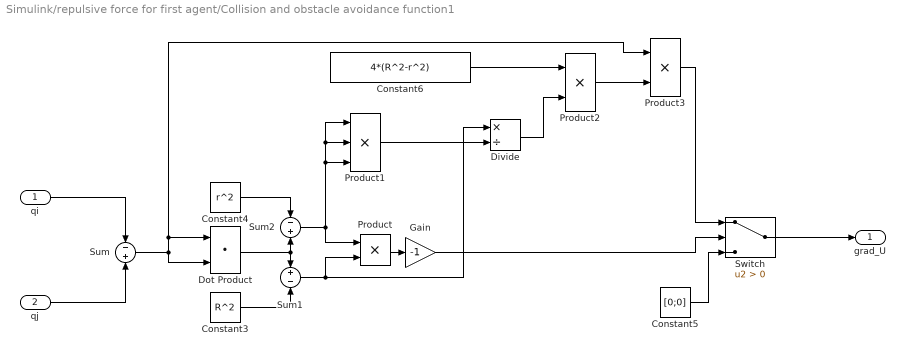
== system Simulink/repulsive force for first agent/Collision and obstacle avoidance function1 ==
  qi : Inport
  qj : Inport  Port=2
  Constant3 : Constant  Value=R^2
  Constant4 : Constant  Value=r^2
  Constant5 : Constant  Value=[0;0]
  Constant6 : Constant  Value=4*(R^2-r^2)
  Divide : Product  Inputs=*/
  Dot Product : DotProduct  InputSameDT=on  OutDataTypeStr=Inherit: Inherit via internal rule
  Gain : Gain  Gain=-1
  Product : Product
  Product1 : Product  Inputs=3
  Product2 : Product
  Product3 : Product
  Sum : Sum  Inputs=-+
  Sum1 : Sum  Inputs=+-
  Sum2 : Sum  Inputs=-+
  Switch : Switch  Criteria=u2 > Threshold
  grad_U : Outport
  wires:
  qj/1 -> Sum/2
  Switch/1 -> grad_U/1
  Product2/1 -> Product3/2
  Product3/1 -> Switch/1
  Constant6/1 -> Product2/1
  Gain/1 -> Switch/2
  Product/1 -> Gain/1
  Sum/1 -> Dot Product/2, Dot Product/1, Product3/1
  Constant3/1 -> Sum1/2
  Divide/1 -> Product2/2
  Constant4/1 -> Sum2/1
  Constant5/1 -> Switch/3
  Product1/1 -> Divide/2
  Dot Product/1 -> Sum1/1, Sum2/2
  qi/1 -> Sum/1
  Sum2/1 -> Product/1, Product1/3, Product1/2, Product1/1
  Sum1/1 -> Product/2, Divide/1
